simulink model "test_feedbackWithDelay"  (R2023b)
settings: Solver=VariableStepAuto  StartTime=0.0  StopTime=10.0  RelTol=1e-3
values from neighbouring files (symbols this model uses):
  nDelay = ceil(350*.25)    [Laser_n_PID_initializer.m]    (also in bode_check_stability_w_time_delay.m = 319)
  s = estimate_iir_transfer_function(x,y,3,1)    [linearModelization.m]
libraries: slctrl_linear x3, simulink x1
settings Model: Creator=lastline  LastModifiedBy=lastline

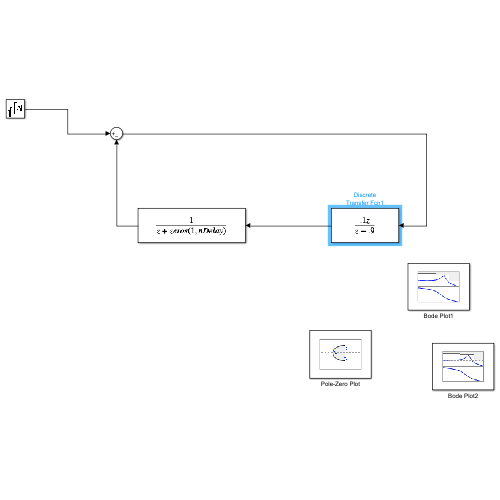
[thumbnail: Simulink's stored preview of the top-level diagram]
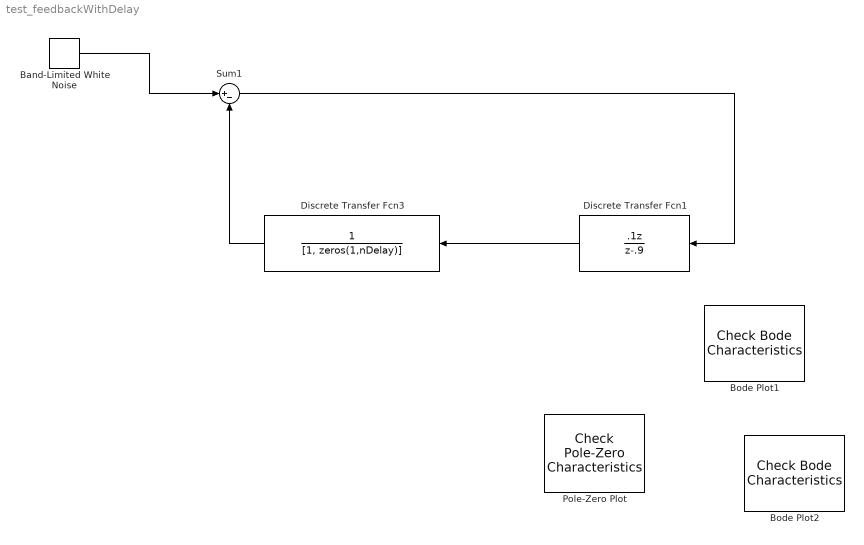
== system test_feedbackWithDelay ==
  Band-Limited White Noise : simulink/Sources/Band-Limited White Noise  Cov=[0.1]  Ts=0.1  seed=[23341]
  Bode Plot1 : slctrl_linear/Check Bode  Characteristics  InstantiateOnLoad=on  SaveOperatingPoints=off  LinearizationIOs={'/Band-Limited White Noise', 1, 'in', 'off', '';'/Sum1', 1, 'out', 'off', ''}  LinearizeAt=SnapshotTimes  SnapshotTimes=[0]  TriggerType=rising  SampleTime=auto  RateConversionMethod=zoh  PreWarpFreq=10  UseExactDelayModel=off  UseFullBlockNameLabels=off  UseBusSignalLabels=off  enabled=on  stopWhenAssertionFail=off  export=off  ViewDlgPos=[1 80 1920 924]  OpenViewOnLoad=on  LaunchViewOnOpen=on  FrequencyUnits=rad/s  MagnitudeUnits=dB  PhaseUnits=deg  TimeUnits=seconds  EnableUpperBound=off  UpperBoundFrequencies=[]  UpperBoundMagnitudes=[]  EnableLowerBound=off  LowerBoundFrequencies=[]  LowerBoundMagnitudes=[]
      settings: LibrarySourceBlock=slctrlblks/Linear Analysis Plots/Bode Plot  SaveToWorkspace=off  SaveName=sys
  Bode Plot2 : slctrl_linear/Check Bode  Characteristics  InstantiateOnLoad=on  SaveOperatingPoints=off  LinearizationIOs={'/Band-Limited White Noise', 1, 'in', 'off', '';'/Discrete Transfer Fcn1', 1, 'out', 'on', ''}  LinearizeAt=SnapshotTimes  SnapshotTimes=[0]  TriggerType=rising  SampleTime=auto  RateConversionMethod=zoh  PreWarpFreq=10  UseExactDelayModel=off  UseFullBlockNameLabels=off  UseBusSignalLabels=off  enabled=on  stopWhenAssertionFail=off  export=off  ViewDlgPos=[1 80 1920 924]  OpenViewOnLoad=on  LaunchViewOnOpen=on  FrequencyUnits=rad/s  MagnitudeUnits=dB  PhaseUnits=deg  TimeUnits=seconds  EnableUpperBound=off  UpperBoundFrequencies=[]  UpperBoundMagnitudes=[]  EnableLowerBound=off  LowerBoundFrequencies=[]  LowerBoundMagnitudes=[]
      settings: LibrarySourceBlock=slctrlblks/Linear Analysis Plots/Bode Plot  SaveToWorkspace=off  SaveName=sys
  Discrete Transfer Fcn1 : DiscreteTransferFcn  Numerator=[.1 0]  Denominator=[1 -.9]
  Discrete Transfer Fcn3 : DiscreteTransferFcn  Denominator=[1, zeros(1,nDelay)]  a0EqualsOne=on
  Pole-Zero Plot : slctrl_linear/Check Pole-Zero Characteristics  InstantiateOnLoad=on  SaveOperatingPoints=off  LinearizationIOs={'/Band-Limited White Noise', 1, 'in', 'off', '';'/Sum1', 1, 'out', 'off', ''}  LinearizeAt=SnapshotTimes  SnapshotTimes=[0]  TriggerType=rising  SampleTime=auto  RateConversionMethod=zoh  PreWarpFreq=10  UseExactDelayModel=off  UseFullBlockNameLabels=off  UseBusSignalLabels=off  enabled=on  stopWhenAssertionFail=off  export=off  ViewDlgPos=[2050 14 916 888]  LaunchViewOnOpen=on  OpenViewOnLoad=on  FrequencyUnits=rad/s  MagnitudeUnits=dB  PhaseUnits=deg  TimeUnits=seconds  EnableSettlingTime=off  SettlingTime=[]  EnablePercentOvershoot=off  PercentOvershoot=[]  EnableDampingRatio=off  DampingRatio=[]  EnableNaturalFrequency=off  NaturalFrequencyBound=>=  NaturalFrequency=[]
      settings: LibrarySourceBlock=slctrlblks/Linear Analysis Plots/Pole-Zero Plot  SaveToWorkspace=off  SaveName=sys
  Sum1 : Sum  Inputs=|+-
  wires:
  Band-Limited White Noise/1 -> Sum1/1
  Discrete Transfer Fcn3/1 -> Sum1/2
  Sum1/1 -> Discrete Transfer Fcn1/1
  Discrete Transfer Fcn1/1 -> Discrete Transfer Fcn3/1
